simulink model "c00014M_harness"  (R2018a)
settings: Solver=FixedStepAuto  StartTime=0.0  StopTime=300  FixedStep=0.1  RelTol=1e-3
undefined symbols (not defined in the file): A1, hmax, PriorityTank, R1, R2, sigbuilder_block
(part 1 of 24)
settings Model: Creator=aarrieta  LastModifiedBy=umarkiegi

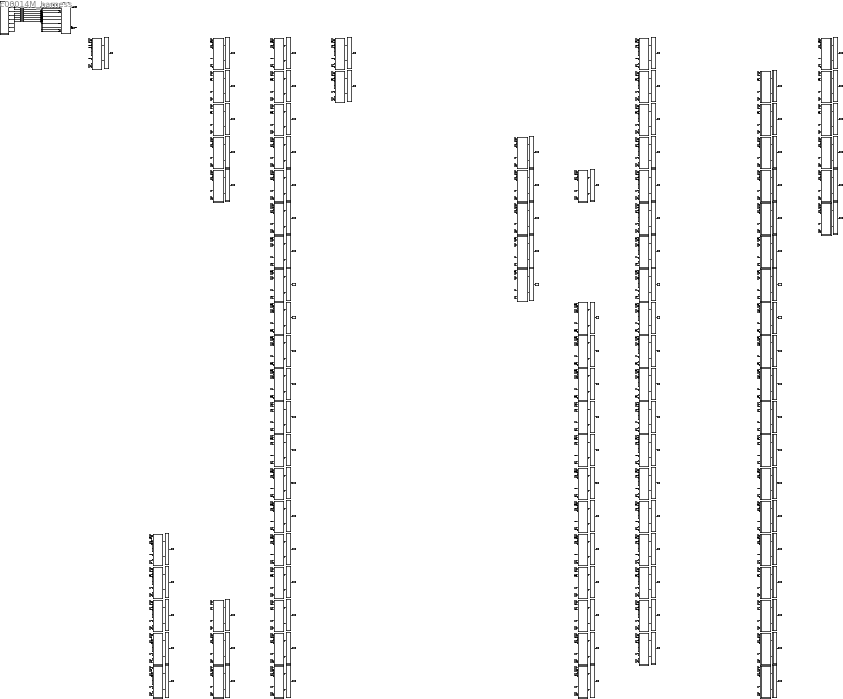
== system c00014M_harness ==
  CPSUT : Subsystem
  Eval : Subsystem
  Eval143 : Subsystem
  Eval144 : Subsystem
  Eval145 : Subsystem
  Eval146 : Subsystem
  Eval147 : Subsystem
  Eval164 : Subsystem
  Eval168 : Subsystem
  Eval169 : Subsystem
  Eval170 : Subsystem
  Eval171 : Subsystem
  Eval172 : Subsystem
  Eval173 : Subsystem
  Eval174 : Subsystem
  Eval175 : Subsystem
  Eval176 : Subsystem
  Eval177 : Subsystem
  Eval178 : Subsystem
  Eval179 : Subsystem
  Eval180 : Subsystem
  Eval181 : Subsystem
  Eval182 : Subsystem
  Eval183 : Subsystem
  Eval184 : Subsystem
  Eval185 : Subsystem
  Eval186 : Subsystem
  Eval187 : Subsystem
  Eval188 : Subsystem
  Eval189 : Subsystem
  Eval190 : Subsystem
  Eval191 : Subsystem
  Eval192 : Subsystem
  Eval193 : Subsystem
  Eval194 : Subsystem
  Eval195 : Subsystem
  Eval196 : Subsystem
  Eval197 : Subsystem
  Eval198 : Subsystem
  Eval221 : Subsystem
  Eval222 : Subsystem
  Eval223 : Subsystem
  Eval224 : Subsystem
  Eval225 : Subsystem
  Eval226 : Subsystem
  Eval227 : Subsystem
  Eval228 : Subsystem
  Eval229 : Subsystem
  Eval230 : Subsystem
  Eval231 : Subsystem
  Eval232 : Subsystem
  Eval233 : Subsystem
  Eval234 : Subsystem
  Eval235 : Subsystem
  Eval236 : Subsystem
  Eval237 : Subsystem
  Eval238 : Subsystem
  Eval239 : Subsystem
  Eval240 : Subsystem
  Eval241 : Subsystem
  Eval242 : Subsystem
  Eval243 : Subsystem
  Eval244 : Subsystem
  Eval245 : Subsystem
  Eval35 : Subsystem
  Eval36 : Subsystem
  Eval37 : Subsystem
  Eval38 : Subsystem
  Eval39 : Subsystem
  Eval40 : Subsystem
  Eval41 : Subsystem
  Eval42 : Subsystem
  Eval43 : Subsystem
  Eval44 : Subsystem
  Eval57 : Subsystem
  Eval58 : Subsystem
  Eval59 : Subsystem
  Eval60 : Subsystem
  Eval61 : Subsystem
  Eval62 : Subsystem
  Eval63 : Subsystem
  Eval64 : Subsystem
  Eval65 : Subsystem
  Eval66 : Subsystem
  Eval67 : Subsystem
  Eval68 : Subsystem
  Eval69 : Subsystem
  Eval70 : Subsystem
  Eval71 : Subsystem
  Eval72 : Subsystem
  Eval73 : Subsystem
  Eval74 : Subsystem
  Eval75 : Subsystem
  Eval76 : Subsystem
  Eval77 : Subsystem
  Eval78 : Subsystem
  Eval79 : Subsystem
  Eval80 : Subsystem
  Eval81 : Subsystem
  Inputs : Subsystem  Tag=STV Subsys  LoadFcn=sigbuilder_block('load');  StartFcn=sigbuilder_block('start');  StopFcn=sigbuilder_block('stop');  ClipboardFcn=sigbuilder_block('clipboard');  mask(Sigbuilder block){tuvar=[0:10]}
      mask init:
      | if ~strcmp(get_param(bdroot(gcb),'SimulationStatus'),'stopped'),tuvar = sigbuilder_block('maskInit'); end
      settings: CopyFcn=sigbuilder_block('copy');  DeleteFcn=sigbuilder_block('delete');  ModelCloseFcn=sigbuilder_block('modelClose');  PreSaveFcn=sigbuilder_block('preSave');  PauseFcn=sigbuilder_block('pause');  ContinueFcn=sigbuilder_block('continue');  NameChangeFcn=sigbuilder_block('namechange');  OpenFcn=sigbuilder_block('open',[276.75 163.5 675.75 486.75 ]);  CloseFcn=sigbuilder_block('close');
      mask Display: plot(0, 0, 100, 100,[2, 2, 32, 32, 2], [68, 8, 8, 68, 68],[32, 2], [38, 38], [32, 19, 2],[53, 60, 44], [32, 17, 17, 2],[16, 16, 31, 31]);txt = getActiveGroup(gcbh);text(2, 100, txt,'verticalAlignment', 'top');
  M001 : Subsystem
  M036 : Subsystem
  M037 : Subsystem
  M038 : Subsystem
  M039 : Subsystem
  M040 : Subsystem
  M041 : Subsystem
  M042 : Subsystem
  M043 : Subsystem
  M044 : Subsystem
  M045 : Subsystem
  M058 : Subsystem
  M059 : Subsystem
  M060 : Subsystem
  M061 : Subsystem
  M062 : Subsystem
  M063 : Subsystem
  M064 : Subsystem
  M065 : Subsystem
  M066 : Subsystem
  M067 : Subsystem
  M068 : Subsystem
  M069 : Subsystem
  M070 : Subsystem
  M071 : Subsystem
  M072 : Subsystem
  M073 : Subsystem
  M074 : Subsystem
  M075 : Subsystem
  M076 : Subsystem
  M077 : Subsystem
  M078 : Subsystem
  M079 : Subsystem
  M080 : Subsystem
  M081 : Subsystem
  M082 : Subsystem
  M144 : Subsystem
  M145 : Subsystem
  M146 : Subsystem
  M147 : Subsystem
  M148 : Subsystem
  M165 : Subsystem
  M169 : Subsystem
  M170 : Subsystem
  M171 : Subsystem
  M172 : Subsystem
  M173 : Subsystem
  M174 : Subsystem
  M175 : Subsystem
  M176 : Subsystem
  M177 : Subsystem
  M178 : Subsystem
  M179 : Subsystem
  M180 : Subsystem
  M181 : Subsystem
  M182 : Subsystem
  M183 : Subsystem
  M184 : Subsystem
  M185 : Subsystem
  M186 : Subsystem
  M187 : Subsystem
  M188 : Subsystem
  M189 : Subsystem
  M190 : Subsystem
  M191 : Subsystem
  M192 : Subsystem
  M193 : Subsystem
  M194 : Subsystem
  M195 : Subsystem
  M196 : Subsystem
  M197 : Subsystem
  M198 : Subsystem
  M199 : Subsystem
  M222 : Subsystem
  M223 : Subsystem
  M224 : Subsystem
  M225 : Subsystem
  M226 : Subsystem
  M227 : Subsystem
  M228 : Subsystem
  M229 : Subsystem
  M230 : Subsystem
  M231 : Subsystem
  M232 : Subsystem
  M233 : Subsystem
  M234 : Subsystem
  M235 : Subsystem
  M236 : Subsystem
  M237 : Subsystem
  M238 : Subsystem
  M239 : Subsystem
  M240 : Subsystem
  M241 : Subsystem
  M242 : Subsystem
  M243 : Subsystem
  M244 : Subsystem
  M245 : Subsystem
  M246 : Subsystem
  To Workspace : ToWorkspace  VariableName=mutant001  SampleTime=-1
  To Workspace143 : ToWorkspace  VariableName=mutant144  SampleTime=-1
  To Workspace144 : ToWorkspace  VariableName=mutant145  SampleTime=-1
  To Workspace145 : ToWorkspace  VariableName=mutant146  SampleTime=-1
  To Workspace146 : ToWorkspace  VariableName=mutant147  SampleTime=-1
  To Workspace147 : ToWorkspace  VariableName=mutant148  SampleTime=-1
  To Workspace164 : ToWorkspace  VariableName=mutant165  SampleTime=-1
  To Workspace168 : ToWorkspace  VariableName=mutant169  SampleTime=-1
  To Workspace169 : ToWorkspace  VariableName=mutant170  SampleTime=-1
  To Workspace170 : ToWorkspace  VariableName=mutant171  SampleTime=-1
  To Workspace171 : ToWorkspace  VariableName=mutant172  SampleTime=-1
  To Workspace172 : ToWorkspace  VariableName=mutant173  SampleTime=-1
  To Workspace173 : ToWorkspace  VariableName=mutant174  SampleTime=-1
  To Workspace174 : ToWorkspace  VariableName=mutant175  SampleTime=-1
  To Workspace175 : ToWorkspace  VariableName=mutant176  SampleTime=-1
  To Workspace176 : ToWorkspace  VariableName=mutant177  SampleTime=-1
  To Workspace177 : ToWorkspace  VariableName=mutant178  SampleTime=-1
  To Workspace178 : ToWorkspace  VariableName=mutant179  SampleTime=-1
  To Workspace179 : ToWorkspace  VariableName=mutant180  SampleTime=-1
  To Workspace180 : ToWorkspace  VariableName=mutant181  SampleTime=-1
  To Workspace181 : ToWorkspace  VariableName=mutant182  SampleTime=-1
  To Workspace182 : ToWorkspace  VariableName=mutant183  SampleTime=-1
  To Workspace183 : ToWorkspace  VariableName=mutant184  SampleTime=-1
  To Workspace184 : ToWorkspace  VariableName=mutant185  SampleTime=-1
  To Workspace185 : ToWorkspace  VariableName=mutant186  SampleTime=-1
  To Workspace186 : ToWorkspace  VariableName=mutant187  SampleTime=-1
  To Workspace187 : ToWorkspace  VariableName=mutant188  SampleTime=-1
  To Workspace188 : ToWorkspace  VariableName=mutant189  SampleTime=-1
  To Workspace189 : ToWorkspace  VariableName=mutant190  SampleTime=-1
  To Workspace190 : ToWorkspace  VariableName=mutant191  SampleTime=-1
  To Workspace191 : ToWorkspace  VariableName=mutant192  SampleTime=-1
  To Workspace192 : ToWorkspace  VariableName=mutant193  SampleTime=-1
  To Workspace193 : ToWorkspace  VariableName=mutant194  SampleTime=-1
  To Workspace194 : ToWorkspace  VariableName=mutant195  SampleTime=-1
  To Workspace195 : ToWorkspace  VariableName=mutant196  SampleTime=-1
  To Workspace196 : ToWorkspace  VariableName=mutant197  SampleTime=-1
  To Workspace197 : ToWorkspace  VariableName=mutant198  SampleTime=-1
  To Workspace198 : ToWorkspace  VariableName=mutant199  SampleTime=-1
  To Workspace221 : ToWorkspace  VariableName=mutant222  SampleTime=-1
  To Workspace222 : ToWorkspace  VariableName=mutant223  SampleTime=-1
  To Workspace223 : ToWorkspace  VariableName=mutant224  SampleTime=-1
  To Workspace224 : ToWorkspace  VariableName=mutant225  SampleTime=-1
  To Workspace225 : ToWorkspace  VariableName=mutant226  SampleTime=-1
  To Workspace226 : ToWorkspace  VariableName=mutant227  SampleTime=-1
  To Workspace227 : ToWorkspace  VariableName=mutant228  SampleTime=-1
  To Workspace228 : ToWorkspace  VariableName=mutant229  SampleTime=-1
  To Workspace229 : ToWorkspace  VariableName=mutant230  SampleTime=-1
  To Workspace230 : ToWorkspace  VariableName=mutant231  SampleTime=-1
  To Workspace231 : ToWorkspace  VariableName=mutant232  SampleTime=-1
  To Workspace232 : ToWorkspace  VariableName=mutant233  SampleTime=-1
  To Workspace233 : ToWorkspace  VariableName=mutant234  SampleTime=-1
  To Workspace234 : ToWorkspace  VariableName=mutant235  SampleTime=-1
  To Workspace235 : ToWorkspace  VariableName=mutant236  SampleTime=-1
  To Workspace236 : ToWorkspace  VariableName=mutant237  SampleTime=-1
  To Workspace237 : ToWorkspace  VariableName=mutant238  SampleTime=-1
  To Workspace238 : ToWorkspace  VariableName=mutant239  SampleTime=-1
  To Workspace239 : ToWorkspace  VariableName=mutant240  SampleTime=-1
  To Workspace240 : ToWorkspace  VariableName=mutant241  SampleTime=-1
  To Workspace241 : ToWorkspace  VariableName=mutant242  SampleTime=-1
  To Workspace242 : ToWorkspace  VariableName=mutant243  SampleTime=-1
  To Workspace243 : ToWorkspace  VariableName=mutant244  SampleTime=-1
  To Workspace244 : ToWorkspace  VariableName=mutant245  SampleTime=-1
  To Workspace245 : ToWorkspace  VariableName=mutant246  SampleTime=-1
  To Workspace35 : ToWorkspace  VariableName=mutant036  SampleTime=-1
  To Workspace36 : ToWorkspace  VariableName=mutant037  SampleTime=-1
  To Workspace37 : ToWorkspace  VariableName=mutant038  SampleTime=-1
  To Workspace38 : ToWorkspace  VariableName=mutant039  SampleTime=-1
  To Workspace39 : ToWorkspace  VariableName=mutant040  SampleTime=-1
  To Workspace40 : ToWorkspace  VariableName=mutant041  SampleTime=-1
  To Workspace41 : ToWorkspace  VariableName=mutant042  SampleTime=-1
  To Workspace42 : ToWorkspace  VariableName=mutant043  SampleTime=-1
  To Workspace43 : ToWorkspace  VariableName=mutant044  SampleTime=-1
  To Workspace44 : ToWorkspace  VariableName=mutant045  SampleTime=-1
  To Workspace57 : ToWorkspace  VariableName=mutant058  SampleTime=-1
  To Workspace58 : ToWorkspace  VariableName=mutant059  SampleTime=-1
  To Workspace59 : ToWorkspace  VariableName=mutant060  SampleTime=-1
  To Workspace60 : ToWorkspace  VariableName=mutant061  SampleTime=-1
  To Workspace61 : ToWorkspace  VariableName=mutant062  SampleTime=-1
  To Workspace62 : ToWorkspace  VariableName=mutant063  SampleTime=-1
  To Workspace63 : ToWorkspace  VariableName=mutant064  SampleTime=-1
  To Workspace64 : ToWorkspace  VariableName=mutant065  SampleTime=-1
  To Workspace65 : ToWorkspace  VariableName=mutant066  SampleTime=-1
  To Workspace66 : ToWorkspace  VariableName=mutant067  SampleTime=-1
  To Workspace67 : ToWorkspace  VariableName=mutant068  SampleTime=-1
  To Workspace68 : ToWorkspace  VariableName=mutant069  SampleTime=-1
  To Workspace69 : ToWorkspace  VariableName=mutant070  SampleTime=-1
  To Workspace70 : ToWorkspace  VariableName=mutant071  SampleTime=-1
  To Workspace71 : ToWorkspace  VariableName=mutant072  SampleTime=-1
  To Workspace72 : ToWorkspace  VariableName=mutant073  SampleTime=-1
  To Workspace73 : ToWorkspace  VariableName=mutant074  SampleTime=-1
  To Workspace74 : ToWorkspace  VariableName=mutant075  SampleTime=-1
  To Workspace75 : ToWorkspace  VariableName=mutant076  SampleTime=-1
  To Workspace76 : ToWorkspace  VariableName=mutant077  SampleTime=-1
  To Workspace77 : ToWorkspace  VariableName=mutant078  SampleTime=-1
  To Workspace78 : ToWorkspace  VariableName=mutant079  SampleTime=-1
  To Workspace79 : ToWorkspace  VariableName=mutant080  SampleTime=-1
  To Workspace80 : ToWorkspace  VariableName=mutant081  SampleTime=-1
  To Workspace81 : ToWorkspace  VariableName=mutant082  SampleTime=-1
  dtc_CT1 : DataTypeConversion
  dtc_CT3 : DataTypeConversion
  dtc_E1 : DataTypeConversion
  dtc_EB1 : DataTypeConversion
  dtc_EB3 : DataTypeConversion
  dtc_F1 : DataTypeConversion
  dtc_T1 : DataTypeConversion
  dtc_T3 : DataTypeConversion
  LL1 : Outport
  LL3 : Outport  Port=2
  tag scope: out1=global, out3=global
  wires:
  CPSUT/1(LL1) -> [out1], LL1/1
  CPSUT/2(LL3) -> [out3], LL3/1
  [in1] -> M001/1(CT1)
  [in2] -> M001/2(F1)
  [in3] -> M001/3(E1)
  [in5] -> M001/4(T1)
  [in6] -> M001/5(EB1)
  [in13] -> M001/6(CT3)
  [in17] -> M001/7(T3)
  [in18] -> M001/8(EB3)
  Eval/1(Out1) -> To Workspace/1
  M001/1(LL1) -> Eval/1(In1)
  M001/2(LL3) -> Eval/2(In3)
  [in1] -> M036/1(CT1)
  [in2] -> M036/2(F1)
  [in3] -> M036/3(E1)
  [in5] -> M036/4(T1)
  [in6] -> M036/5(EB1)
  [in13] -> M036/6(CT3)
  [in17] -> M036/7(T3)
  [in18] -> M036/8(EB3)
  M036/1(LL1) -> Eval35/1(In1)
  M036/2(LL3) -> Eval35/2(In3)
  Eval35/1(Out1) -> To Workspace35/1
  [in1] -> M037/1(CT1)
  [in2] -> M037/2(F1)
  [in3] -> M037/3(E1)
  [in5] -> M037/4(T1)
  [in6] -> M037/5(EB1)
  [in13] -> M037/6(CT3)
  [in17] -> M037/7(T3)
  [in18] -> M037/8(EB3)
  M037/1(LL1) -> Eval36/1(In1)
  M037/2(LL3) -> Eval36/2(In3)
  Eval36/1(Out1) -> To Workspace36/1
  [in1] -> M038/1(CT1)
  [in2] -> M038/2(F1)
  [in3] -> M038/3(E1)
  [in5] -> M038/4(T1)
  [in6] -> M038/5(EB1)
  [in13] -> M038/6(CT3)
  [in17] -> M038/7(T3)
  [in18] -> M038/8(EB3)
  M038/1(LL1) -> Eval37/1(In1)
  M038/2(LL3) -> Eval37/2(In3)
  Eval37/1(Out1) -> To Workspace37/1
  [in1] -> M039/1(CT1)
  [in2] -> M039/2(F1)
  [in3] -> M039/3(E1)
  [in5] -> M039/4(T1)
  [in6] -> M039/5(EB1)
  [in13] -> M039/6(CT3)
  [in17] -> M039/7(T3)
  [in18] -> M039/8(EB3)
  M039/1(LL1) -> Eval38/1(In1)
  M039/2(LL3) -> Eval38/2(In3)
  Eval38/1(Out1) -> To Workspace38/1
  [in1] -> M040/1(CT1)
  [in2] -> M040/2(F1)
  [in3] -> M040/3(E1)
  [in5] -> M040/4(T1)
  [in6] -> M040/5(EB1)
  [in13] -> M040/6(CT3)
  [in17] -> M040/7(T3)
  [in18] -> M040/8(EB3)
  M040/1(LL1) -> Eval39/1(In1)
  M040/2(LL3) -> Eval39/2(In3)
  Eval39/1(Out1) -> To Workspace39/1
  [in1] -> M041/1(CT1)
  [in2] -> M041/2(F1)
  [in3] -> M041/3(E1)
  [in5] -> M041/4(T1)
  [in6] -> M041/5(EB1)
  [in13] -> M041/6(CT3)
  [in17] -> M041/7(T3)
  [in18] -> M041/8(EB3)
  M041/1(LL1) -> Eval40/1(In1)
  M041/2(LL3) -> Eval40/2(In3)
  Eval40/1(Out1) -> To Workspace40/1
  [in1] -> M042/1(CT1)
  [in2] -> M042/2(F1)
  [in3] -> M042/3(E1)
  [in5] -> M042/4(T1)
  [in6] -> M042/5(EB1)
  [in13] -> M042/6(CT3)
  [in17] -> M042/7(T3)
  [in18] -> M042/8(EB3)
  M042/1(LL1) -> Eval41/1(In1)
  M042/2(LL3) -> Eval41/2(In3)
  Eval41/1(Out1) -> To Workspace41/1
  [in1] -> M043/1(CT1)
  [in2] -> M043/2(F1)
  [in3] -> M043/3(E1)
  [in5] -> M043/4(T1)
  [in6] -> M043/5(EB1)
  [in13] -> M043/6(CT3)
  [in17] -> M043/7(T3)
  [in18] -> M043/8(EB3)
  M043/1(LL1) -> Eval42/1(In1)
  M043/2(LL3) -> Eval42/2(In3)
  Eval42/1(Out1) -> To Workspace42/1
  [in1] -> M044/1(CT1)
  [in2] -> M044/2(F1)
  [in3] -> M044/3(E1)
  [in5] -> M044/4(T1)
  [in6] -> M044/5(EB1)
  [in13] -> M044/6(CT3)
  [in17] -> M044/7(T3)
  [in18] -> M044/8(EB3)
  M044/1(LL1) -> Eval43/1(In1)
  M044/2(LL3) -> Eval43/2(In3)
  Eval43/1(Out1) -> To Workspace43/1
  [in1] -> M045/1(CT1)
  [in2] -> M045/2(F1)
  [in3] -> M045/3(E1)
  [in5] -> M045/4(T1)
  [in6] -> M045/5(EB1)
  [in13] -> M045/6(CT3)
  [in17] -> M045/7(T3)
  [in18] -> M045/8(EB3)
  M045/1(LL1) -> Eval44/1(In1)
  M045/2(LL3) -> Eval44/2(In3)
  Eval44/1(Out1) -> To Workspace44/1
  [in1] -> M058/1(CT1)
  [in2] -> M058/2(F1)
  [in3] -> M058/3(E1)
  [in5] -> M058/4(T1)
  [in6] -> M058/5(EB1)
  [in13] -> M058/6(CT3)
  [in17] -> M058/7(T3)
  [in18] -> M058/8(EB3)
  M058/1(LL1) -> Eval57/1(In1)
  M058/2(LL3) -> Eval57/2(In3)
  Eval57/1(Out1) -> To Workspace57/1
  [in1] -> M059/1(CT1)
  [in2] -> M059/2(F1)
  [in3] -> M059/3(E1)
  [in5] -> M059/4(T1)
  [in6] -> M059/5(EB1)
  [in13] -> M059/6(CT3)
  [in17] -> M059/7(T3)
  [in18] -> M059/8(EB3)
  M059/1(LL1) -> Eval58/1(In1)
  M059/2(LL3) -> Eval58/2(In3)
  Eval58/1(Out1) -> To Workspace58/1
  [in1] -> M060/1(CT1)
  [in2] -> M060/2(F1)
  [in3] -> M060/3(E1)
  [in5] -> M060/4(T1)
  [in6] -> M060/5(EB1)
  [in13] -> M060/6(CT3)
  [in17] -> M060/7(T3)
  [in18] -> M060/8(EB3)
  M060/1(LL1) -> Eval59/1(In1)
  M060/2(LL3) -> Eval59/2(In3)
  Eval59/1(Out1) -> To Workspace59/1
  [in1] -> M061/1(CT1)
  [in2] -> M061/2(F1)
  [in3] -> M061/3(E1)
  [in5] -> M061/4(T1)
  [in6] -> M061/5(EB1)
  [in13] -> M061/6(CT3)
  [in17] -> M061/7(T3)
  [in18] -> M061/8(EB3)
  M061/1(LL1) -> Eval60/1(In1)
  M061/2(LL3) -> Eval60/2(In3)
  Eval60/1(Out1) -> To Workspace60/1
  [in1] -> M062/1(CT1)
  [in2] -> M062/2(F1)
  [in3] -> M062/3(E1)
  [in5] -> M062/4(T1)
  [in6] -> M062/5(EB1)
  [in13] -> M062/6(CT3)
  [in17] -> M062/7(T3)
  [in18] -> M062/8(EB3)
  M062/1(LL1) -> Eval61/1(In1)
  M062/2(LL3) -> Eval61/2(In3)
  Eval61/1(Out1) -> To Workspace61/1
  [in1] -> M063/1(CT1)
  [in2] -> M063/2(F1)
  [in3] -> M063/3(E1)
  [in5] -> M063/4(T1)
  [in6] -> M063/5(EB1)
  [in13] -> M063/6(CT3)
  [in17] -> M063/7(T3)
  [in18] -> M063/8(EB3)
  M063/1(LL1) -> Eval62/1(In1)
  M063/2(LL3) -> Eval62/2(In3)
  Eval62/1(Out1) -> To Workspace62/1
  [in1] -> M064/1(CT1)
  [in2] -> M064/2(F1)
  [in3] -> M064/3(E1)
  [in5] -> M064/4(T1)
  [in6] -> M064/5(EB1)
  [in13] -> M064/6(CT3)
  [in17] -> M064/7(T3)
  [in18] -> M064/8(EB3)
  M064/1(LL1) -> Eval63/1(In1)
  M064/2(LL3) -> Eval63/2(In3)
  Eval63/1(Out1) -> To Workspace63/1
  [in1] -> M065/1(CT1)
  [in2] -> M065/2(F1)
  [in3] -> M065/3(E1)
  [in5] -> M065/4(T1)
  [in6] -> M065/5(EB1)
  [in13] -> M065/6(CT3)
  [in17] -> M065/7(T3)
  [in18] -> M065/8(EB3)
  M065/1(LL1) -> Eval64/1(In1)
  M065/2(LL3) -> Eval64/2(In3)
  Eval64/1(Out1) -> To Workspace64/1
  [in1] -> M066/1(CT1)
  [in2] -> M066/2(F1)
  [in3] -> M066/3(E1)
  [in5] -> M066/4(T1)
  [in6] -> M066/5(EB1)
  [in13] -> M066/6(CT3)
  [in17] -> M066/7(T3)
  [in18] -> M066/8(EB3)
  M066/1(LL1) -> Eval65/1(In1)
  M066/2(LL3) -> Eval65/2(In3)
  Eval65/1(Out1) -> To Workspace65/1
  [in1] -> M067/1(CT1)
  [in2] -> M067/2(F1)
  [in3] -> M067/3(E1)
  [in5] -> M067/4(T1)
  [in6] -> M067/5(EB1)
  [in13] -> M067/6(CT3)
  [in17] -> M067/7(T3)
  [in18] -> M067/8(EB3)
  M067/1(LL1) -> Eval66/1(In1)
  M067/2(LL3) -> Eval66/2(In3)
  Eval66/1(Out1) -> To Workspace66/1
  [in1] -> M068/1(CT1)
  [in2] -> M068/2(F1)
  [in3] -> M068/3(E1)
  [in5] -> M068/4(T1)
  [in6] -> M068/5(EB1)
  [in13] -> M068/6(CT3)
  [in17] -> M068/7(T3)
  [in18] -> M068/8(EB3)
  M068/1(LL1) -> Eval67/1(In1)
  M068/2(LL3) -> Eval67/2(In3)
  Eval67/1(Out1) -> To Workspace67/1
  [in1] -> M069/1(CT1)
  [in2] -> M069/2(F1)
  [in3] -> M069/3(E1)
  [in5] -> M069/4(T1)
  [in6] -> M069/5(EB1)
  [in13] -> M069/6(CT3)
  [in17] -> M069/7(T3)
  [in18] -> M069/8(EB3)
  M069/1(LL1) -> Eval68/1(In1)
  M069/2(LL3) -> Eval68/2(In3)
  Eval68/1(Out1) -> To Workspace68/1
  [in1] -> M070/1(CT1)
  [in2] -> M070/2(F1)
  [in3] -> M070/3(E1)
  [in5] -> M070/4(T1)
  [in6] -> M070/5(EB1)
  [in13] -> M070/6(CT3)
  [in17] -> M070/7(T3)
  [in18] -> M070/8(EB3)
  M070/1(LL1) -> Eval69/1(In1)
  M070/2(LL3) -> Eval69/2(In3)
  Eval69/1(Out1) -> To Workspace69/1
  [in1] -> M071/1(CT1)
  [in2] -> M071/2(F1)
  [in3] -> M071/3(E1)
  [in5] -> M071/4(T1)
  [in6] -> M071/5(EB1)
  [in13] -> M071/6(CT3)
  [in17] -> M071/7(T3)
  [in18] -> M071/8(EB3)
  M071/1(LL1) -> Eval70/1(In1)
  M071/2(LL3) -> Eval70/2(In3)
  Eval70/1(Out1) -> To Workspace70/1
  [in1] -> M072/1(CT1)
  [in2] -> M072/2(F1)
  [in3] -> M072/3(E1)
  [in5] -> M072/4(T1)
  [in6] -> M072/5(EB1)
  [in13] -> M072/6(CT3)
  [in17] -> M072/7(T3)
  [in18] -> M072/8(EB3)
  M072/1(LL1) -> Eval71/1(In1)
  M072/2(LL3) -> Eval71/2(In3)
  Eval71/1(Out1) -> To Workspace71/1
  [in1] -> M073/1(CT1)
  [in2] -> M073/2(F1)
  [in3] -> M073/3(E1)
  [in5] -> M073/4(T1)
  [in6] -> M073/5(EB1)
  [in13] -> M073/6(CT3)
  [in17] -> M073/7(T3)
  [in18] -> M073/8(EB3)
  M073/1(LL1) -> Eval72/1(In1)
  M073/2(LL3) -> Eval72/2(In3)
  Eval72/1(Out1) -> To Workspace72/1
  [in1] -> M074/1(CT1)
  [in2] -> M074/2(F1)
  [in3] -> M074/3(E1)
  [in5] -> M074/4(T1)
  [in6] -> M074/5(EB1)
  [in13] -> M074/6(CT3)
  [in17] -> M074/7(T3)
  [in18] -> M074/8(EB3)
  M074/1(LL1) -> Eval73/1(In1)
  M074/2(LL3) -> Eval73/2(In3)
  Eval73/1(Out1) -> To Workspace73/1
  [in1] -> M075/1(CT1)
  [in2] -> M075/2(F1)
  [in3] -> M075/3(E1)
  [in5] -> M075/4(T1)
  [in6] -> M075/5(EB1)
  [in13] -> M075/6(CT3)
  [in17] -> M075/7(T3)
  [in18] -> M075/8(EB3)
  M075/1(LL1) -> Eval74/1(In1)
  M075/2(LL3) -> Eval74/2(In3)
  Eval74/1(Out1) -> To Workspace74/1
  [in1] -> M076/1(CT1)
  [in2] -> M076/2(F1)
  [in3] -> M076/3(E1)
  [in5] -> M076/4(T1)
  [in6] -> M076/5(EB1)
  [in13] -> M076/6(CT3)
  [in17] -> M076/7(T3)
  [in18] -> M076/8(EB3)
  M076/1(LL1) -> Eval75/1(In1)
  M076/2(LL3) -> Eval75/2(In3)
  Eval75/1(Out1) -> To Workspace75/1
  [in1] -> M077/1(CT1)
  [in2] -> M077/2(F1)
  [in3] -> M077/3(E1)
  [in5] -> M077/4(T1)
  [in6] -> M077/5(EB1)
  [in13] -> M077/6(CT3)
  [in17] -> M077/7(T3)
  [in18] -> M077/8(EB3)
  M077/1(LL1) -> Eval76/1(In1)
  M077/2(LL3) -> Eval76/2(In3)
  Eval76/1(Out1) -> To Workspace76/1
  [in1] -> M078/1(CT1)
  [in2] -> M078/2(F1)
  [in3] -> M078/3(E1)
  [in5] -> M078/4(T1)
  [in6] -> M078/5(EB1)
  [in13] -> M078/6(CT3)
  [in17] -> M078/7(T3)
  [in18] -> M078/8(EB3)
  M078/1(LL1) -> Eval77/1(In1)
  M078/2(LL3) -> Eval77/2(In3)
  Eval77/1(Out1) -> To Workspace77/1
  [in1] -> M079/1(CT1)
  [in2] -> M079/2(F1)
  [in3] -> M079/3(E1)
  [in5] -> M079/4(T1)
  [in6] -> M079/5(EB1)
  [in13] -> M079/6(CT3)
  [in17] -> M079/7(T3)
  [in18] -> M079/8(EB3)
  M079/1(LL1) -> Eval78/1(In1)
  M079/2(LL3) -> Eval78/2(In3)
  Eval78/1(Out1) -> To Workspace78/1
  [in1] -> M080/1(CT1)
  [in2] -> M080/2(F1)
  [in3] -> M080/3(E1)
  [in5] -> M080/4(T1)
  [in6] -> M080/5(EB1)
  [in13] -> M080/6(CT3)
  [in17] -> M080/7(T3)
  [in18] -> M080/8(EB3)
  M080/1(LL1) -> Eval79/1(In1)
  M080/2(LL3) -> Eval79/2(In3)
  Eval79/1(Out1) -> To Workspace79/1
  [in1] -> M081/1(CT1)
  [in2] -> M081/2(F1)
  [in3] -> M081/3(E1)
  [in5] -> M081/4(T1)
  [in6] -> M081/5(EB1)
  [in13] -> M081/6(CT3)
  [in17] -> M081/7(T3)
  [in18] -> M081/8(EB3)
  M081/1(LL1) -> Eval80/1(In1)
  M081/2(LL3) -> Eval80/2(In3)
  Eval80/1(Out1) -> To Workspace80/1
  [in1] -> M082/1(CT1)
  [in2] -> M082/2(F1)
  [in3] -> M082/3(E1)
  [in5] -> M082/4(T1)
  [in6] -> M082/5(EB1)
  [in13] -> M082/6(CT3)
  [in17] -> M082/7(T3)
  [in18] -> M082/8(EB3)
  M082/1(LL1) -> Eval81/1(In1)
  M082/2(LL3) -> Eval81/2(In3)
  Eval81/1(Out1) -> To Workspace81/1
  [in1] -> M144/1(CT1)
  [in2] -> M144/2(F1)
  [in3] -> M144/3(E1)
  [in5] -> M144/4(T1)
  [in6] -> M144/5(EB1)
  [in13] -> M144/6(CT3)
  [in17] -> M144/7(T3)
  [in18] -> M144/8(EB3)
  M144/1(LL1) -> Eval143/1(In1)
  M144/2(LL3) -> Eval143/2(In3)
  Eval143/1(Out1) -> To Workspace143/1
  [in1] -> M145/1(CT1)
  [in2] -> M145/2(F1)
  [in3] -> M145/3(E1)
  [in5] -> M145/4(T1)
  [in6] -> M145/5(EB1)
  [in13] -> M145/6(CT3)
  [in17] -> M145/7(T3)
  [in18] -> M145/8(EB3)
  M145/1(LL1) -> Eval144/1(In1)
  M145/2(LL3) -> Eval144/2(In3)
  Eval144/1(Out1) -> To Workspace144/1
  [in1] -> M146/1(CT1)
  [in2] -> M146/2(F1)
  [in3] -> M146/3(E1)
  [in5] -> M146/4(T1)
  [in6] -> M146/5(EB1)
  [in13] -> M146/6(CT3)
  [in17] -> M146/7(T3)
  [in18] -> M146/8(EB3)
  M146/1(LL1) -> Eval145/1(In1)
  M146/2(LL3) -> Eval145/2(In3)
  Eval145/1(Out1) -> To Workspace145/1
  [in1] -> M147/1(CT1)
  [in2] -> M147/2(F1)
  [in3] -> M147/3(E1)
  [in5] -> M147/4(T1)
  [in6] -> M147/5(EB1)
  [in13] -> M147/6(CT3)
  [in17] -> M147/7(T3)
  [in18] -> M147/8(EB3)
  M147/1(LL1) -> Eval146/1(In1)
  M147/2(LL3) -> Eval146/2(In3)
  Eval146/1(Out1) -> To Workspace146/1
  [in1] -> M148/1(CT1)
  [in2] -> M148/2(F1)
  [in3] -> M148/3(E1)
  [in5] -> M148/4(T1)
  [in6] -> M148/5(EB1)
  [in13] -> M148/6(CT3)
  [in17] -> M148/7(T3)
  [in18] -> M148/8(EB3)
  M148/1(LL1) -> Eval147/1(In1)
  M148/2(LL3) -> Eval147/2(In3)
  Eval147/1(Out1) -> To Workspace147/1
  [in1] -> M165/1(CT1)
  [in2] -> M165/2(F1)
  [in3] -> M165/3(E1)
  [in5] -> M165/4(T1)
  [in6] -> M165/5(EB1)
  [in13] -> M165/6(CT3)
  [in17] -> M165/7(T3)
  [in18] -> M165/8(EB3)
  M165/1(LL1) -> Eval164/1(In1)
  M165/2(LL3) -> Eval164/2(In3)
  Eval164/1(Out1) -> To Workspace164/1
  [in1] -> M169/1(CT1)
  [in2] -> M169/2(F1)
  [in3] -> M169/3(E1)
  [in5] -> M169/4(T1)
  [in6] -> M169/5(EB1)
  [in13] -> M169/6(CT3)
  [in17] -> M169/7(T3)
  [in18] -> M169/8(EB3)
  M169/1(LL1) -> Eval168/1(In1)
  M169/2(LL3) -> Eval168/2(In3)
  Eval168/1(Out1) -> To Workspace168/1
  [in1] -> M170/1(CT1)
  [in2] -> M170/2(F1)
  [in3] -> M170/3(E1)
  [in5] -> M170/4(T1)
  [in6] -> M170/5(EB1)
  [in13] -> M170/6(CT3)
  [in17] -> M170/7(T3)
  [in18] -> M170/8(EB3)
  M170/1(LL1) -> Eval169/1(In1)
  M170/2(LL3) -> Eval169/2(In3)
  Eval169/1(Out1) -> To Workspace169/1
  [in1] -> M171/1(CT1)
  [in2] -> M171/2(F1)
  [in3] -> M171/3(E1)
  [in5] -> M171/4(T1)
  [in6] -> M171/5(EB1)
  [in13] -> M171/6(CT3)
  [in17] -> M171/7(T3)
  [in18] -> M171/8(EB3)
  M171/1(LL1) -> Eval170/1(In1)
  M171/2(LL3) -> Eval170/2(In3)
  Eval170/1(Out1) -> To Workspace170/1
  [in1] -> M172/1(CT1)
  [in2] -> M172/2(F1)
  [in3] -> M172/3(E1)
  [in5] -> M172/4(T1)
  [in6] -> M172/5(EB1)
  [in13] -> M172/6(CT3)
  [in17] -> M172/7(T3)
  [in18] -> M172/8(EB3)
  M172/1(LL1) -> Eval171/1(In1)
  M172/2(LL3) -> Eval171/2(In3)
  Eval171/1(Out1) -> To Workspace171/1
  [in1] -> M173/1(CT1)
  [in2] -> M173/2(F1)
  [in3] -> M173/3(E1)
  [in5] -> M173/4(T1)
  [in6] -> M173/5(EB1)
  [in13] -> M173/6(CT3)
  [in17] -> M173/7(T3)
  [in18] -> M173/8(EB3)
  M173/1(LL1) -> Eval172/1(In1)
  M173/2(LL3) -> Eval172/2(In3)
  Eval172/1(Out1) -> To Workspace172/1
  [in1] -> M174/1(CT1)
  [in2] -> M174/2(F1)
  [in3] -> M174/3(E1)
  [in5] -> M174/4(T1)
  [in6] -> M174/5(EB1)
  [in13] -> M174/6(CT3)
  [in17] -> M174/7(T3)
  [in18] -> M174/8(EB3)
  M174/1(LL1) -> Eval173/1(In1)
  M174/2(LL3) -> Eval173/2(In3)
  Eval173/1(Out1) -> To Workspace173/1
  [in1] -> M175/1(CT1)
  [in2] -> M175/2(F1)
  [in3] -> M175/3(E1)
  [in5] -> M175/4(T1)
  [in6] -> M175/5(EB1)
  [in13] -> M175/6(CT3)
  [in17] -> M175/7(T3)
  [in18] -> M175/8(EB3)
  M175/1(LL1) -> Eval174/1(In1)
  M175/2(LL3) -> Eval174/2(In3)
  Eval174/1(Out1) -> To Workspace174/1
  [in1] -> M176/1(CT1)
  [in2] -> M176/2(F1)
  [in3] -> M176/3(E1)
  [in5] -> M176/4(T1)
  [in6] -> M176/5(EB1)
  [in13] -> M176/6(CT3)
  [in17] -> M176/7(T3)
  [in18] -> M176/8(EB3)
  M176/1(LL1) -> Eval175/1(In1)
  M176/2(LL3) -> Eval175/2(In3)
  Eval175/1(Out1) -> To Workspace175/1
  [in1] -> M177/1(CT1)
  [in2] -> M177/2(F1)
  [in3] -> M177/3(E1)
  [in5] -> M177/4(T1)
  [in6] -> M177/5(EB1)
  [in13] -> M177/6(CT3)
  [in17] -> M177/7(T3)
  [in18] -> M177/8(EB3)
  M177/1(LL1) -> Eval176/1(In1)
  M177/2(LL3) -> Eval176/2(In3)
  Eval176/1(Out1) -> To Workspace176/1
  [in1] -> M178/1(CT1)
  [in2] -> M178/2(F1)
  [in3] -> M178/3(E1)
  [in5] -> M178/4(T1)
  [in6] -> M178/5(EB1)
  [in13] -> M178/6(CT3)
  [in17] -> M178/7(T3)
  [in18] -> M178/8(EB3)
  M178/1(LL1) -> Eval177/1(In1)
  M178/2(LL3) -> Eval177/2(In3)
  Eval177/1(Out1) -> To Workspace177/1
  [in1] -> M179/1(CT1)
  [in2] -> M179/2(F1)
  [in3] -> M179/3(E1)
  [in5] -> M179/4(T1)
  [in6] -> M179/5(EB1)
  [in13] -> M179/6(CT3)
  [in17] -> M179/7(T3)
  [in18] -> M179/8(EB3)
  M179/1(LL1) -> Eval178/1(In1)
  M179/2(LL3) -> Eval178/2(In3)
  Eval178/1(Out1) -> To Workspace178/1
  [in1] -> M180/1(CT1)
  [in2] -> M180/2(F1)
  [in3] -> M180/3(E1)
  [in5] -> M180/4(T1)
  [in6] -> M180/5(EB1)
  [in13] -> M180/6(CT3)
  [in17] -> M180/7(T3)
  [in18] -> M180/8(EB3)
  M180/1(LL1) -> Eval179/1(In1)
  M180/2(LL3) -> Eval179/2(In3)
  Eval179/1(Out1) -> To Workspace179/1
  [in1] -> M181/1(CT1)
  [in2] -> M181/2(F1)
  [in3] -> M181/3(E1)
  [in5] -> M181/4(T1)
  [in6] -> M181/5(EB1)
  [in13] -> M181/6(CT3)
  [in17] -> M181/7(T3)
  [in18] -> M181/8(EB3)
  M181/1(LL1) -> Eval180/1(In1)
  M181/2(LL3) -> Eval180/2(In3)
  Eval180/1(Out1) -> To Workspace180/1
  [in1] -> M182/1(CT1)
  [in2] -> M182/2(F1)
  [in3] -> M182/3(E1)
  [in5] -> M182/4(T1)
  [in6] -> M182/5(EB1)
  [in13] -> M182/6(CT3)
  [in17] -> M182/7(T3)
  [in18] -> M182/8(EB3)
  M182/1(LL1) -> Eval181/1(In1)
  M182/2(LL3) -> Eval181/2(In3)
  Eval181/1(Out1) -> To Workspace181/1
  [in1] -> M183/1(CT1)
  [in2] -> M183/2(F1)
  [in3] -> M183/3(E1)
  [in5] -> M183/4(T1)
  [in6] -> M183/5(EB1)
  [in13] -> M183/6(CT3)
  [in17] -> M183/7(T3)
  [in18] -> M183/8(EB3)
  M183/1(LL1) -> Eval182/1(In1)
  M183/2(LL3) -> Eval182/2(In3)
  Eval182/1(Out1) -> To Workspace182/1
  [in1] -> M184/1(CT1)
  [in2] -> M184/2(F1)
  [in3] -> M184/3(E1)
  [in5] -> M184/4(T1)
  [in6] -> M184/5(EB1)
  [in13] -> M184/6(CT3)
  [in17] -> M184/7(T3)
  [in18] -> M184/8(EB3)
  M184/1(LL1) -> Eval183/1(In1)
  M184/2(LL3) -> Eval183/2(In3)
  Eval183/1(Out1) -> To Workspace183/1
  [in1] -> M185/1(CT1)
  [in2] -> M185/2(F1)
  [in3] -> M185/3(E1)
  [in5] -> M185/4(T1)
  [in6] -> M185/5(EB1)
  [in13] -> M185/6(CT3)
  [in17] -> M185/7(T3)
  [in18] -> M185/8(EB3)
  M185/1(LL1) -> Eval184/1(In1)
  M185/2(LL3) -> Eval184/2(In3)
  Eval184/1(Out1) -> To Workspace184/1
  [in1] -> M186/1(CT1)
  [in2] -> M186/2(F1)
  [in3] -> M186/3(E1)
  [in5] -> M186/4(T1)
  [in6] -> M186/5(EB1)
  [in13] -> M186/6(CT3)
  [in17] -> M186/7(T3)
  [in18] -> M186/8(EB3)
  M186/1(LL1) -> Eval185/1(In1)
  M186/2(LL3) -> Eval185/2(In3)
  Eval185/1(Out1) -> To Workspace185/1
  [in1] -> M187/1(CT1)
  [in2] -> M187/2(F1)
  [in3] -> M187/3(E1)
  [in5] -> M187/4(T1)
  [in6] -> M187/5(EB1)
  [in13] -> M187/6(CT3)
  [in17] -> M187/7(T3)
  [in18] -> M187/8(EB3)
  M187/1(LL1) -> Eval186/1(In1)
  M187/2(LL3) -> Eval186/2(In3)
  Eval186/1(Out1) -> To Workspace186/1
  [in1] -> M188/1(CT1)
  [in2] -> M188/2(F1)
  [in3] -> M188/3(E1)
  [in5] -> M188/4(T1)
  [in6] -> M188/5(EB1)
  [in13] -> M188/6(CT3)
  [in17] -> M188/7(T3)
  [in18] -> M188/8(EB3)
  M188/1(LL1) -> Eval187/1(In1)
  M188/2(LL3) -> Eval187/2(In3)
  Eval187/1(Out1) -> To Workspace187/1
  [in1] -> M189/1(CT1)
  [in2] -> M189/2(F1)
  [in3] -> M189/3(E1)
  [in5] -> M189/4(T1)
  [in6] -> M189/5(EB1)
  [in13] -> M189/6(CT3)
  [in17] -> M189/7(T3)
  [in18] -> M189/8(EB3)
  M189/1(LL1) -> Eval188/1(In1)
  M189/2(LL3) -> Eval188/2(In3)
  Eval188/1(Out1) -> To Workspace188/1
  [in1] -> M190/1(CT1)
  [in2] -> M190/2(F1)
  [in3] -> M190/3(E1)
  [in5] -> M190/4(T1)
  [in6] -> M190/5(EB1)
  [in13] -> M190/6(CT3)
  [in17] -> M190/7(T3)
  [in18] -> M190/8(EB3)
  M190/1(LL1) -> Eval189/1(In1)
  M190/2(LL3) -> Eval189/2(In3)
  Eval189/1(Out1) -> To Workspace189/1
  [in1] -> M191/1(CT1)
  [in2] -> M191/2(F1)
  [in3] -> M191/3(E1)
  [in5] -> M191/4(T1)
  [in6] -> M191/5(EB1)
  [in13] -> M191/6(CT3)
  [in17] -> M191/7(T3)
  [in18] -> M191/8(EB3)
  M191/1(LL1) -> Eval190/1(In1)
  M191/2(LL3) -> Eval190/2(In3)
  Eval190/1(Out1) -> To Workspace190/1
  [in1] -> M192/1(CT1)
  [in2] -> M192/2(F1)
  [in3] -> M192/3(E1)
  [in5] -> M192/4(T1)
  [in6] -> M192/5(EB1)
  [in13] -> M192/6(CT3)
  [in17] -> M192/7(T3)
  [in18] -> M192/8(EB3)
  M192/1(LL1) -> Eval191/1(In1)
  M192/2(LL3) -> Eval191/2(In3)
  Eval191/1(Out1) -> To Workspace191/1
  [in1] -> M193/1(CT1)
  [in2] -> M193/2(F1)
  [in3] -> M193/3(E1)
  [in5] -> M193/4(T1)
  [in6] -> M193/5(EB1)
  [in13] -> M193/6(CT3)
  [in17] -> M193/7(T3)
  [in18] -> M193/8(EB3)
  M193/1(LL1) -> Eval192/1(In1)
  M193/2(LL3) -> Eval192/2(In3)
  Eval192/1(Out1) -> To Workspace192/1
  [in1] -> M194/1(CT1)
  [in2] -> M194/2(F1)
  [in3] -> M194/3(E1)
  [in5] -> M194/4(T1)
  [in6] -> M194/5(EB1)
  [in13] -> M194/6(CT3)
  [in17] -> M194/7(T3)
  [in18] -> M194/8(EB3)
  M194/1(LL1) -> Eval193/1(In1)
  M194/2(LL3) -> Eval193/2(In3)
  Eval193/1(Out1) -> To Workspace193/1
  [in1] -> M195/1(CT1)
  [in2] -> M195/2(F1)
  [in3] -> M195/3(E1)
  [in5] -> M195/4(T1)
  [in6] -> M195/5(EB1)
  [in13] -> M195/6(CT3)
  [in17] -> M195/7(T3)
  [in18] -> M195/8(EB3)
  M195/1(LL1) -> Eval194/1(In1)
  M195/2(LL3) -> Eval194/2(In3)
  Eval194/1(Out1) -> To Workspace194/1
  [in1] -> M196/1(CT1)
  [in2] -> M196/2(F1)
  [in3] -> M196/3(E1)
  [in5] -> M196/4(T1)
  [in6] -> M196/5(EB1)
  [in13] -> M196/6(CT3)
  [in17] -> M196/7(T3)
  [in18] -> M196/8(EB3)
  M196/1(LL1) -> Eval195/1(In1)
  M196/2(LL3) -> Eval195/2(In3)
  Eval195/1(Out1) -> To Workspace195/1
  [in1] -> M197/1(CT1)
  [in2] -> M197/2(F1)
  [in3] -> M197/3(E1)
  [in5] -> M197/4(T1)
  [in6] -> M197/5(EB1)
  [in13] -> M197/6(CT3)
  [in17] -> M197/7(T3)
  [in18] -> M197/8(EB3)
  M197/1(LL1) -> Eval196/1(In1)
  M197/2(LL3) -> Eval196/2(In3)
  Eval196/1(Out1) -> To Workspace196/1
  [in1] -> M198/1(CT1)
  [in2] -> M198/2(F1)
  [in3] -> M198/3(E1)
  [in5] -> M198/4(T1)
  [in6] -> M198/5(EB1)
  [in13] -> M198/6(CT3)
  [in17] -> M198/7(T3)
  [in18] -> M198/8(EB3)
  M198/1(LL1) -> Eval197/1(In1)
  M198/2(LL3) -> Eval197/2(In3)
  Eval197/1(Out1) -> To Workspace197/1
  [in1] -> M199/1(CT1)
  [in2] -> M199/2(F1)
  [in3] -> M199/3(E1)
  [in5] -> M199/4(T1)
  [in6] -> M199/5(EB1)
  [in13] -> M199/6(CT3)
  [in17] -> M199/7(T3)
  [in18] -> M199/8(EB3)
  M199/1(LL1) -> Eval198/1(In1)
  M199/2(LL3) -> Eval198/2(In3)
  Eval198/1(Out1) -> To Workspace198/1
  [in1] -> M222/1(CT1)
  [in2] -> M222/2(F1)
  [in3] -> M222/3(E1)
  [in5] -> M222/4(T1)
  [in6] -> M222/5(EB1)
  [in13] -> M222/6(CT3)
  [in17] -> M222/7(T3)
  [in18] -> M222/8(EB3)
  M222/1(LL1) -> Eval221/1(In1)
  M222/2(LL3) -> Eval221/2(In3)
  Eval221/1(Out1) -> To Workspace221/1
  [in1] -> M223/1(CT1)
  [in2] -> M223/2(F1)
  [in3] -> M223/3(E1)
  [in5] -> M223/4(T1)
  [in6] -> M223/5(EB1)
  [in13] -> M223/6(CT3)
  [in17] -> M223/7(T3)
  [in18] -> M223/8(EB3)
  M223/1(LL1) -> Eval222/1(In1)
  M223/2(LL3) -> Eval222/2(In3)
  Eval222/1(Out1) -> To Workspace222/1
  [in1] -> M224/1(CT1)
  [in2] -> M224/2(F1)
  [in3] -> M224/3(E1)
  [in5] -> M224/4(T1)
  [in6] -> M224/5(EB1)
  [in13] -> M224/6(CT3)
  [in17] -> M224/7(T3)
  [in18] -> M224/8(EB3)
  M224/1(LL1) -> Eval223/1(In1)
  M224/2(LL3) -> Eval223/2(In3)
  Eval223/1(Out1) -> To Workspace223/1
  [in1] -> M225/1(CT1)
  [in2] -> M225/2(F1)
  [in3] -> M225/3(E1)
  [in5] -> M225/4(T1)
  [in6] -> M225/5(EB1)
  [in13] -> M225/6(CT3)
  [in17] -> M225/7(T3)
  [in18] -> M225/8(EB3)
  M225/1(LL1) -> Eval224/1(In1)
  M225/2(LL3) -> Eval224/2(In3)
  Eval224/1(Out1) -> To Workspace224/1
  [in1] -> M226/1(CT1)
  [in2] -> M226/2(F1)
  [in3] -> M226/3(E1)
  [in5] -> M226/4(T1)
  [in6] -> M226/5(EB1)
  [in13] -> M226/6(CT3)
  [in17] -> M226/7(T3)
  [in18] -> M226/8(EB3)
  M226/1(LL1) -> Eval225/1(In1)
  M226/2(LL3) -> Eval225/2(In3)
  Eval225/1(Out1) -> To Workspace225/1
  [in1] -> M227/1(CT1)
  [in2] -> M227/2(F1)
  [in3] -> M227/3(E1)
  [in5] -> M227/4(T1)
  [in6] -> M227/5(EB1)
  [in13] -> M227/6(CT3)
  [in17] -> M227/7(T3)
  [in18] -> M227/8(EB3)
  M227/1(LL1) -> Eval226/1(In1)
  M227/2(LL3) -> Eval226/2(In3)
  Eval226/1(Out1) -> To Workspace226/1
  [in1] -> M228/1(CT1)
  [in2] -> M228/2(F1)
  [in3] -> M228/3(E1)
  [in5] -> M228/4(T1)
  [in6] -> M228/5(EB1)
  [in13] -> M228/6(CT3)
  [in17] -> M228/7(T3)
  [in18] -> M228/8(EB3)
  M228/1(LL1) -> Eval227/1(In1)
  M228/2(LL3) -> Eval227/2(In3)
  Eval227/1(Out1) -> To Workspace227/1
  [in1] -> M229/1(CT1)
  [in2] -> M229/2(F1)
  [in3] -> M229/3(E1)
  [in5] -> M229/4(T1)
  [in6] -> M229/5(EB1)
  [in13] -> M229/6(CT3)
  [in17] -> M229/7(T3)
  [in18] -> M229/8(EB3)
  M229/1(LL1) -> Eval228/1(In1)
  M229/2(LL3) -> Eval228/2(In3)
  Eval228/1(Out1) -> To Workspace228/1
  [in1] -> M230/1(CT1)
  [in2] -> M230/2(F1)
  [in3] -> M230/3(E1)
  [in5] -> M230/4(T1)
  [in6] -> M230/5(EB1)
  [in13] -> M230/6(CT3)
  [in17] -> M230/7(T3)
  [in18] -> M230/8(EB3)
  M230/1(LL1) -> Eval229/1(In1)
  M230/2(LL3) -> Eval229/2(In3)
  Eval229/1(Out1) -> To Workspace229/1
  [in1] -> M231/1(CT1)
  [in2] -> M231/2(F1)
  [in3] -> M231/3(E1)
  [in5] -> M231/4(T1)
  [in6] -> M231/5(EB1)
  [in13] -> M231/6(CT3)
  [in17] -> M231/7(T3)
  [in18] -> M231/8(EB3)
  M231/1(LL1) -> Eval230/1(In1)
  M231/2(LL3) -> Eval230/2(In3)
  Eval230/1(Out1) -> To Workspace230/1
  [in1] -> M232/1(CT1)
  [in2] -> M232/2(F1)
  [in3] -> M232/3(E1)
  [in5] -> M232/4(T1)
  [in6] -> M232/5(EB1)
  [in13] -> M232/6(CT3)
  [in17] -> M232/7(T3)
  [in18] -> M232/8(EB3)
  M232/1(LL1) -> Eval231/1(In1)
  M232/2(LL3) -> Eval231/2(In3)
  Eval231/1(Out1) -> To Workspace231/1
  [in1] -> M233/1(CT1)
  [in2] -> M233/2(F1)
  [in3] -> M233/3(E1)
  [in5] -> M233/4(T1)
  [in6] -> M233/5(EB1)
  [in13] -> M233/6(CT3)
  [in17] -> M233/7(T3)
  [in18] -> M233/8(EB3)
  M233/1(LL1) -> Eval232/1(In1)
  M233/2(LL3) -> Eval232/2(In3)
  Eval232/1(Out1) -> To Workspace232/1
  [in1] -> M234/1(CT1)
  [in2] -> M234/2(F1)
  [in3] -> M234/3(E1)
  [in5] -> M234/4(T1)
  [in6] -> M234/5(EB1)
  [in13] -> M234/6(CT3)
  [in17] -> M234/7(T3)
  [in18] -> M234/8(EB3)
  M234/1(LL1) -> Eval233/1(In1)
  M234/2(LL3) -> Eval233/2(In3)
  Eval233/1(Out1) -> To Workspace233/1
  [in1] -> M235/1(CT1)
  [in2] -> M235/2(F1)
  [in3] -> M235/3(E1)
  [in5] -> M235/4(T1)
  [in6] -> M235/5(EB1)
  [in13] -> M235/6(CT3)
  [in17] -> M235/7(T3)
  [in18] -> M235/8(EB3)
  M235/1(LL1) -> Eval234/1(In1)
  M235/2(LL3) -> Eval234/2(In3)
  Eval234/1(Out1) -> To Workspace234/1
  [in1] -> M236/1(CT1)
  [in2] -> M236/2(F1)
  [in3] -> M236/3(E1)
  [in5] -> M236/4(T1)
  [in6] -> M236/5(EB1)
  [in13] -> M236/6(CT3)
  [in17] -> M236/7(T3)
  [in18] -> M236/8(EB3)
  M236/1(LL1) -> Eval235/1(In1)
  M236/2(LL3) -> Eval235/2(In3)
  Eval235/1(Out1) -> To Workspace235/1
  [in1] -> M237/1(CT1)
  [in2] -> M237/2(F1)
  [in3] -> M237/3(E1)
  [in5] -> M237/4(T1)
  [in6] -> M237/5(EB1)
  [in13] -> M237/6(CT3)
  [in17] -> M237/7(T3)
  [in18] -> M237/8(EB3)
  M237/1(LL1) -> Eval236/1(In1)
  M237/2(LL3) -> Eval236/2(In3)
  Eval236/1(Out1) -> To Workspace236/1
  [in1] -> M238/1(CT1)
  [in2] -> M238/2(F1)
  [in3] -> M238/3(E1)
  [in5] -> M238/4(T1)
  [in6] -> M238/5(EB1)
  [in13] -> M238/6(CT3)
  [in17] -> M238/7(T3)
  [in18] -> M238/8(EB3)
  M238/1(LL1) -> Eval237/1(In1)
  M238/2(LL3) -> Eval237/2(In3)
  Eval237/1(Out1) -> To Workspace237/1
  [in1] -> M239/1(CT1)
  [in2] -> M239/2(F1)
  [in3] -> M239/3(E1)
  [in5] -> M239/4(T1)
  [in6] -> M239/5(EB1)
  [in13] -> M239/6(CT3)
  [in17] -> M239/7(T3)
  [in18] -> M239/8(EB3)
  M239/1(LL1) -> Eval238/1(In1)
  M239/2(LL3) -> Eval238/2(In3)
  Eval238/1(Out1) -> To Workspace238/1
  [in1] -> M240/1(CT1)
  [in2] -> M240/2(F1)
  [in3] -> M240/3(E1)
  [in5] -> M240/4(T1)
  [in6] -> M240/5(EB1)
  [in13] -> M240/6(CT3)
  [in17] -> M240/7(T3)
  [in18] -> M240/8(EB3)
  M240/1(LL1) -> Eval239/1(In1)
  M240/2(LL3) -> Eval239/2(In3)
  Eval239/1(Out1) -> To Workspace239/1
  [in1] -> M241/1(CT1)
  [in2] -> M241/2(F1)
  [in3] -> M241/3(E1)
  [in5] -> M241/4(T1)
  [in6] -> M241/5(EB1)
  [in13] -> M241/6(CT3)
  [in17] -> M241/7(T3)
  [in18] -> M241/8(EB3)
  M241/1(LL1) -> Eval240/1(In1)
  M241/2(LL3) -> Eval240/2(In3)
  Eval240/1(Out1) -> To Workspace240/1
  [in1] -> M242/1(CT1)
  [in2] -> M242/2(F1)
  [in3] -> M242/3(E1)
  [in5] -> M242/4(T1)
  [in6] -> M242/5(EB1)
  [in13] -> M242/6(CT3)
  [in17] -> M242/7(T3)
  [in18] -> M242/8(EB3)
  M242/1(LL1) -> Eval241/1(In1)
  M242/2(LL3) -> Eval241/2(In3)
  Eval241/1(Out1) -> To Workspace241/1
  [in1] -> M243/1(CT1)
  [in2] -> M243/2(F1)
  [in3] -> M243/3(E1)
  [in5] -> M243/4(T1)
  [in6] -> M243/5(EB1)
  [in13] -> M243/6(CT3)
  [in17] -> M243/7(T3)
  [in18] -> M243/8(EB3)
  M243/1(LL1) -> Eval242/1(In1)
  M243/2(LL3) -> Eval242/2(In3)
  Eval242/1(Out1) -> To Workspace242/1
  [in1] -> M244/1(CT1)
  [in2] -> M244/2(F1)
  [in3] -> M244/3(E1)
  [in5] -> M244/4(T1)
  [in6] -> M244/5(EB1)
  [in13] -> M244/6(CT3)
  [in17] -> M244/7(T3)
  [in18] -> M244/8(EB3)
  M244/1(LL1) -> Eval243/1(In1)
  M244/2(LL3) -> Eval243/2(In3)
  Eval243/1(Out1) -> To Workspace243/1
  [in1] -> M245/1(CT1)
  [in2] -> M245/2(F1)
  [in3] -> M245/3(E1)
  [in5] -> M245/4(T1)
  [in6] -> M245/5(EB1)
  [in13] -> M245/6(CT3)
  [in17] -> M245/7(T3)
  [in18] -> M245/8(EB3)
  M245/1(LL1) -> Eval244/1(In1)
  M245/2(LL3) -> Eval244/2(In3)
  Eval244/1(Out1) -> To Workspace244/1
  [in1] -> M246/1(CT1)
  [in2] -> M246/2(F1)
  [in3] -> M246/3(E1)
  [in5] -> M246/4(T1)
  [in6] -> M246/5(EB1)
  [in13] -> M246/6(CT3)
  [in17] -> M246/7(T3)
  [in18] -> M246/8(EB3)
  M246/1(LL1) -> Eval245/1(In1)
  M246/2(LL3) -> Eval245/2(In3)
  Eval245/1(Out1) -> To Workspace245/1
  Inputs/1(CT1) -> dtc_CT1/1
  dtc_CT1/1 -> CPSUT/1(CT1), [in1]
  Inputs/2(F1) -> dtc_F1/1
  dtc_F1/1 -> CPSUT/2(F1), [in2]
  Inputs/3(E1) -> dtc_E1/1
  dtc_E1/1 -> CPSUT/3(E1), [in3]
  Inputs/4(T1) -> dtc_T1/1
  dtc_T1/1 -> CPSUT/4(T1), [in5]
  Inputs/5(EB1) -> dtc_EB1/1
  dtc_EB1/1 -> CPSUT/5(EB1), [in6]
  Inputs/6(CT3) -> dtc_CT3/1
  dtc_CT3/1 -> CPSUT/6(CT3), [in13]
  Inputs/7(T3) -> dtc_T3/1
  dtc_T3/1 -> CPSUT/7(T3), [in17]
  Inputs/8(EB3) -> dtc_EB3/1
  dtc_EB3/1 -> CPSUT/8(EB3), [in18]

== system c00014M_harness/CPSUT ==
  note: VALUES
      | ---------------------------------
      | ControlType = 1 | 2 | 3
      | FillTank = 0 | 1
      | EmptyTank = 0 | 1
      | ManualReference between 0 and 1
      | Tempreature between 0 and 100
      | EmergencyButton = 0 | 1
      | LiquidLevel between 0 and 1 (hmax)
  note: Inputs For Tank2
  note: NAMES
      | --------------------------------------------
      | CT1 = ControlType Tank 1
      | F1 = Fill Tank 1
      | E1 = Empty Tank 1
      | MR1 = Manual Reference Tank1
      | T1 = Temperature Tank 1
      | EB1 = Emergency Button Tank 1
      | LL1 = Liquid Level 1
  note: Inputs For Tank3
  note: Inputs For Tank1
  CT1 : Inport
  F1 : Inport  Port=2
  E1 : Inport  Port=3
  T1 : Inport  Port=4
  EB1 : Inport  Port=5
  CT3 : Inport  Port=6
  T3 : Inport  Port=7
  EB3 : Inport  Port=8
  Tank1 : Subsystem
  Tank3 : Subsystem
  LL1 : Outport
  LL3 : Outport  Port=2
  wires:
  EB1/1 -> Tank1/5(EB1)
  Tank3/1(LL3) -> LL3/1, Tank1/6(LL3)
  T1/1 -> Tank1/4(T1)
  Tank1/1(LL1) -> LL1/1, Tank3/4(LL1)
  F1/1 -> Tank1/2(F1)
  E1/1 -> Tank1/3(E1)
  CT3/1 -> Tank3/1(CT3)
  EB3/1 -> Tank3/3(EB3)
  T3/1 -> Tank3/2(T3)
  CT1/1 -> Tank1/1(CT1)

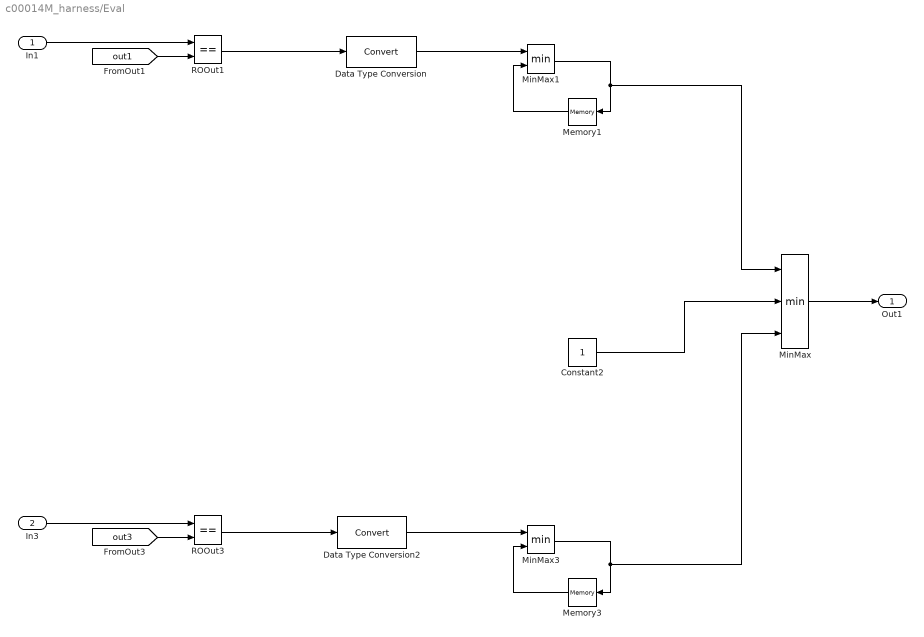
== system c00014M_harness/Eval ==
  In1 : Inport
  In3 : Inport  Port=2
  Constant2 : Constant
  Data Type Conversion : DataTypeConversion
  Data Type Conversion2 : DataTypeConversion
  Memory1 : Memory  InitialCondition=1
  Memory3 : Memory  InitialCondition=1
  MinMax : MinMax  Inputs=3
  MinMax1 : MinMax  Inputs=2
  MinMax3 : MinMax  Inputs=2
  ROOut1 : RelationalOperator  Operator===  OutDataTypeStr=boolean  RndMeth=Simplest
  ROOut3 : RelationalOperator  Operator===  OutDataTypeStr=boolean  RndMeth=Simplest
  Out1 : Outport
  wires:
  MinMax/1 -> Out1/1
  [out3] -> ROOut3/2
  In3/1 -> ROOut3/1
  [out1] -> ROOut1/2
  In1/1 -> ROOut1/1
  Memory1/1 -> MinMax1/2
  MinMax3/1 -> MinMax/3, Memory3/1
  ROOut3/1 -> Data Type Conversion2/1
  Memory3/1 -> MinMax3/2
  ROOut1/1 -> Data Type Conversion/1
  MinMax1/1 -> MinMax/1, Memory1/1
  Data Type Conversion/1 -> MinMax1/1
  Data Type Conversion2/1 -> MinMax3/1
  Constant2/1 -> MinMax/2

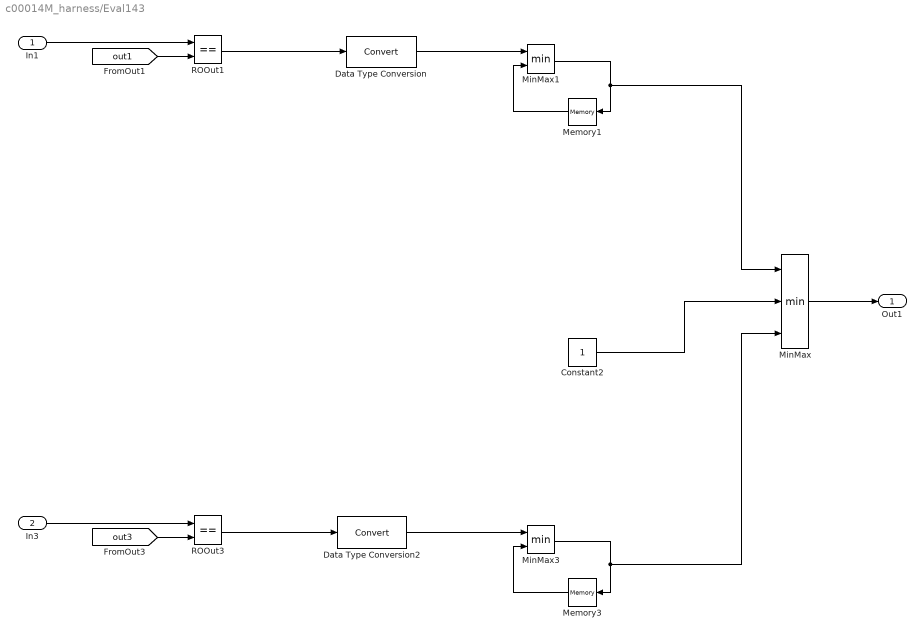
== system c00014M_harness/Eval143 ==
  In1 : Inport
  In3 : Inport  Port=2
  Constant2 : Constant
  Data Type Conversion : DataTypeConversion
  Data Type Conversion2 : DataTypeConversion
  Memory1 : Memory  InitialCondition=1
  Memory3 : Memory  InitialCondition=1
  MinMax : MinMax  Inputs=3
  MinMax1 : MinMax  Inputs=2
  MinMax3 : MinMax  Inputs=2
  ROOut1 : RelationalOperator  Operator===  OutDataTypeStr=boolean  RndMeth=Simplest
  ROOut3 : RelationalOperator  Operator===  OutDataTypeStr=boolean  RndMeth=Simplest
  Out1 : Outport
  wires:
  Data Type Conversion2/1 -> MinMax3/1
  Data Type Conversion/1 -> MinMax1/1
  MinMax1/1 -> Memory1/1, MinMax/1
  ROOut1/1 -> Data Type Conversion/1
  Memory3/1 -> MinMax3/2
  ROOut3/1 -> Data Type Conversion2/1
  MinMax3/1 -> Memory3/1, MinMax/3
  Memory1/1 -> MinMax1/2
  In1/1 -> ROOut1/1
  [out1] -> ROOut1/2
  In3/1 -> ROOut3/1
  [out3] -> ROOut3/2
  MinMax/1 -> Out1/1
  Constant2/1 -> MinMax/2

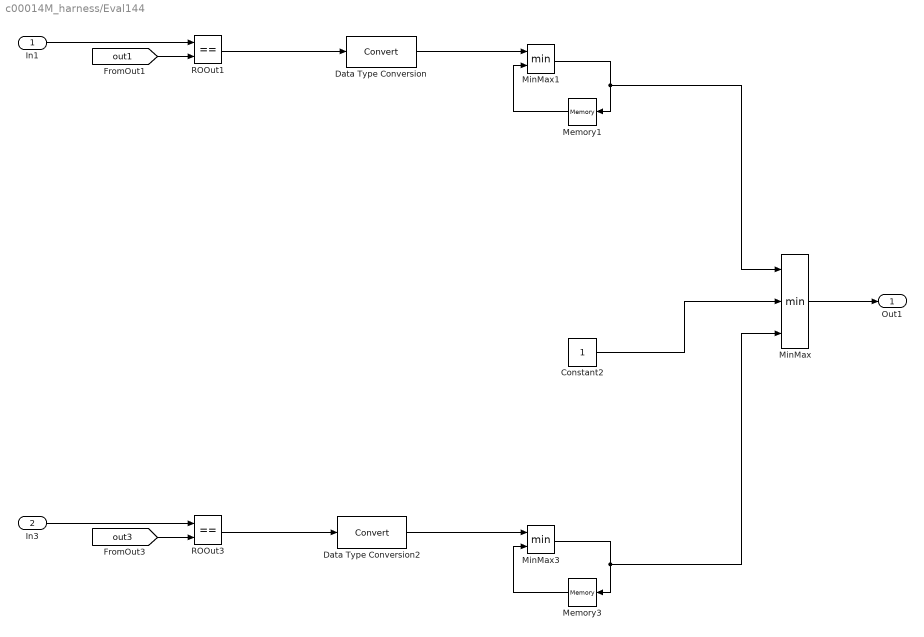
== system c00014M_harness/Eval144 ==
  In1 : Inport
  In3 : Inport  Port=2
  Constant2 : Constant
  Data Type Conversion : DataTypeConversion
  Data Type Conversion2 : DataTypeConversion
  Memory1 : Memory  InitialCondition=1
  Memory3 : Memory  InitialCondition=1
  MinMax : MinMax  Inputs=3
  MinMax1 : MinMax  Inputs=2
  MinMax3 : MinMax  Inputs=2
  ROOut1 : RelationalOperator  Operator===  OutDataTypeStr=boolean  RndMeth=Simplest
  ROOut3 : RelationalOperator  Operator===  OutDataTypeStr=boolean  RndMeth=Simplest
  Out1 : Outport
  wires:
  Data Type Conversion2/1 -> MinMax3/1
  Data Type Conversion/1 -> MinMax1/1
  MinMax1/1 -> Memory1/1, MinMax/1
  ROOut1/1 -> Data Type Conversion/1
  Memory3/1 -> MinMax3/2
  ROOut3/1 -> Data Type Conversion2/1
  MinMax3/1 -> Memory3/1, MinMax/3
  Memory1/1 -> MinMax1/2
  In1/1 -> ROOut1/1
  [out1] -> ROOut1/2
  In3/1 -> ROOut3/1
  [out3] -> ROOut3/2
  MinMax/1 -> Out1/1
  Constant2/1 -> MinMax/2

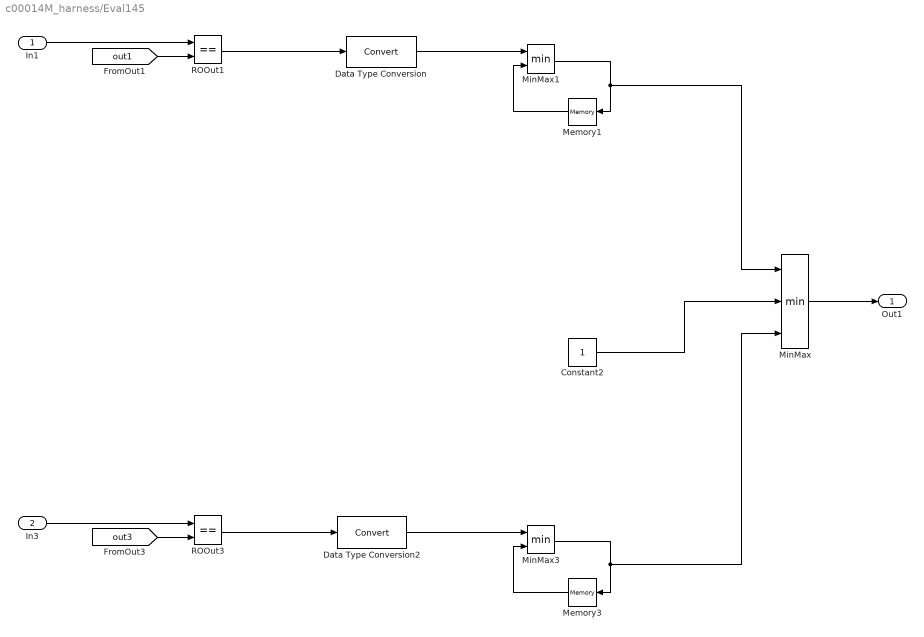
== system c00014M_harness/Eval145 ==
  In1 : Inport
  In3 : Inport  Port=2
  Constant2 : Constant
  Data Type Conversion : DataTypeConversion
  Data Type Conversion2 : DataTypeConversion
  Memory1 : Memory  InitialCondition=1
  Memory3 : Memory  InitialCondition=1
  MinMax : MinMax  Inputs=3
  MinMax1 : MinMax  Inputs=2
  MinMax3 : MinMax  Inputs=2
  ROOut1 : RelationalOperator  Operator===  OutDataTypeStr=boolean  RndMeth=Simplest
  ROOut3 : RelationalOperator  Operator===  OutDataTypeStr=boolean  RndMeth=Simplest
  Out1 : Outport
  wires:
  Data Type Conversion2/1 -> MinMax3/1
  Data Type Conversion/1 -> MinMax1/1
  MinMax1/1 -> Memory1/1, MinMax/1
  ROOut1/1 -> Data Type Conversion/1
  Memory3/1 -> MinMax3/2
  ROOut3/1 -> Data Type Conversion2/1
  MinMax3/1 -> Memory3/1, MinMax/3
  Memory1/1 -> MinMax1/2
  In1/1 -> ROOut1/1
  [out1] -> ROOut1/2
  In3/1 -> ROOut3/1
  [out3] -> ROOut3/2
  MinMax/1 -> Out1/1
  Constant2/1 -> MinMax/2

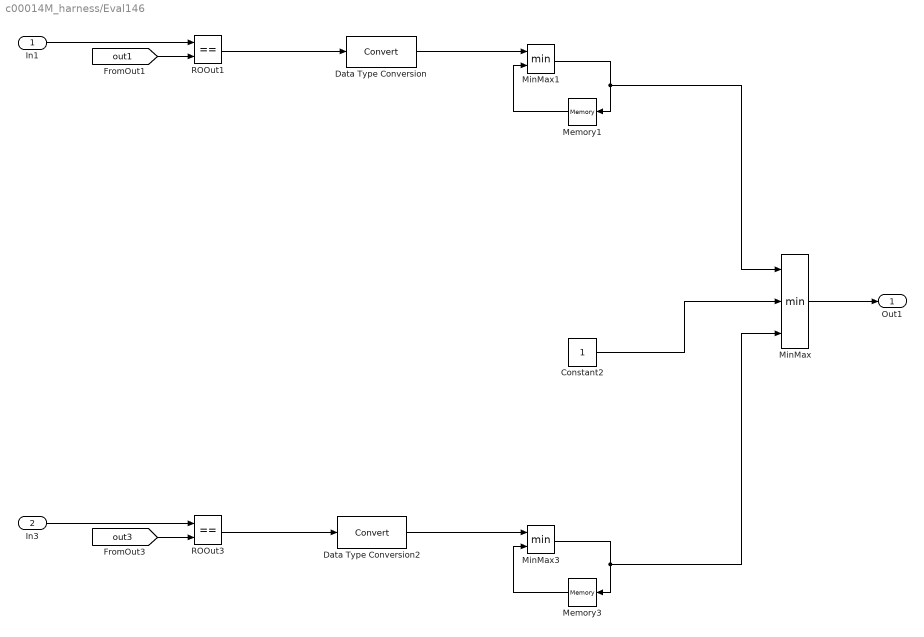
== system c00014M_harness/Eval146 ==
  In1 : Inport
  In3 : Inport  Port=2
  Constant2 : Constant
  Data Type Conversion : DataTypeConversion
  Data Type Conversion2 : DataTypeConversion
  Memory1 : Memory  InitialCondition=1
  Memory3 : Memory  InitialCondition=1
  MinMax : MinMax  Inputs=3
  MinMax1 : MinMax  Inputs=2
  MinMax3 : MinMax  Inputs=2
  ROOut1 : RelationalOperator  Operator===  OutDataTypeStr=boolean  RndMeth=Simplest
  ROOut3 : RelationalOperator  Operator===  OutDataTypeStr=boolean  RndMeth=Simplest
  Out1 : Outport
  wires:
  Data Type Conversion2/1 -> MinMax3/1
  Data Type Conversion/1 -> MinMax1/1
  MinMax1/1 -> Memory1/1, MinMax/1
  ROOut1/1 -> Data Type Conversion/1
  Memory3/1 -> MinMax3/2
  ROOut3/1 -> Data Type Conversion2/1
  MinMax3/1 -> Memory3/1, MinMax/3
  Memory1/1 -> MinMax1/2
  In1/1 -> ROOut1/1
  [out1] -> ROOut1/2
  In3/1 -> ROOut3/1
  [out3] -> ROOut3/2
  MinMax/1 -> Out1/1
  Constant2/1 -> MinMax/2

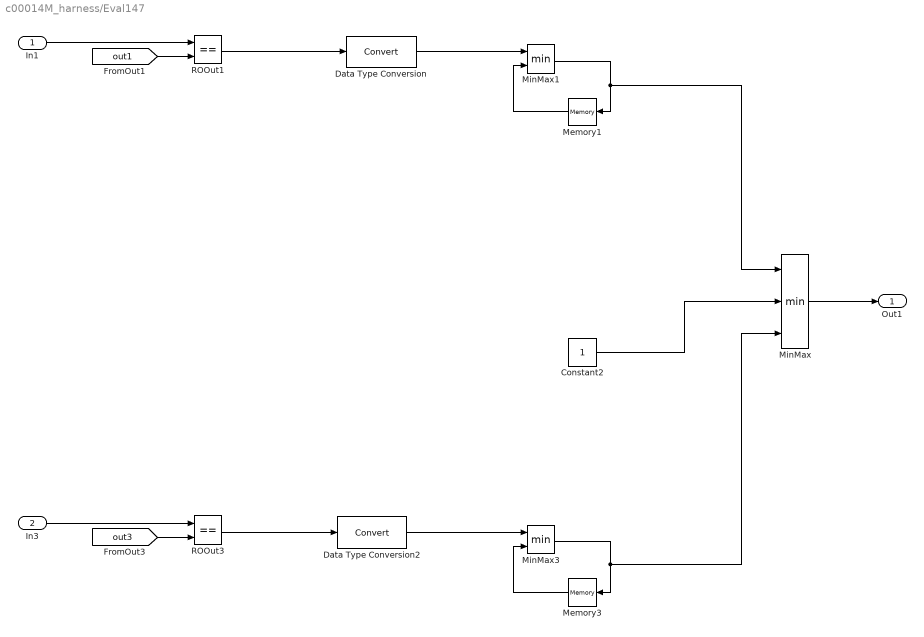
== system c00014M_harness/Eval147 ==
  In1 : Inport
  In3 : Inport  Port=2
  Constant2 : Constant
  Data Type Conversion : DataTypeConversion
  Data Type Conversion2 : DataTypeConversion
  Memory1 : Memory  InitialCondition=1
  Memory3 : Memory  InitialCondition=1
  MinMax : MinMax  Inputs=3
  MinMax1 : MinMax  Inputs=2
  MinMax3 : MinMax  Inputs=2
  ROOut1 : RelationalOperator  Operator===  OutDataTypeStr=boolean  RndMeth=Simplest
  ROOut3 : RelationalOperator  Operator===  OutDataTypeStr=boolean  RndMeth=Simplest
  Out1 : Outport
  wires:
  Data Type Conversion2/1 -> MinMax3/1
  Data Type Conversion/1 -> MinMax1/1
  MinMax1/1 -> Memory1/1, MinMax/1
  ROOut1/1 -> Data Type Conversion/1
  Memory3/1 -> MinMax3/2
  ROOut3/1 -> Data Type Conversion2/1
  MinMax3/1 -> Memory3/1, MinMax/3
  Memory1/1 -> MinMax1/2
  In1/1 -> ROOut1/1
  [out1] -> ROOut1/2
  In3/1 -> ROOut3/1
  [out3] -> ROOut3/2
  MinMax/1 -> Out1/1
  Constant2/1 -> MinMax/2

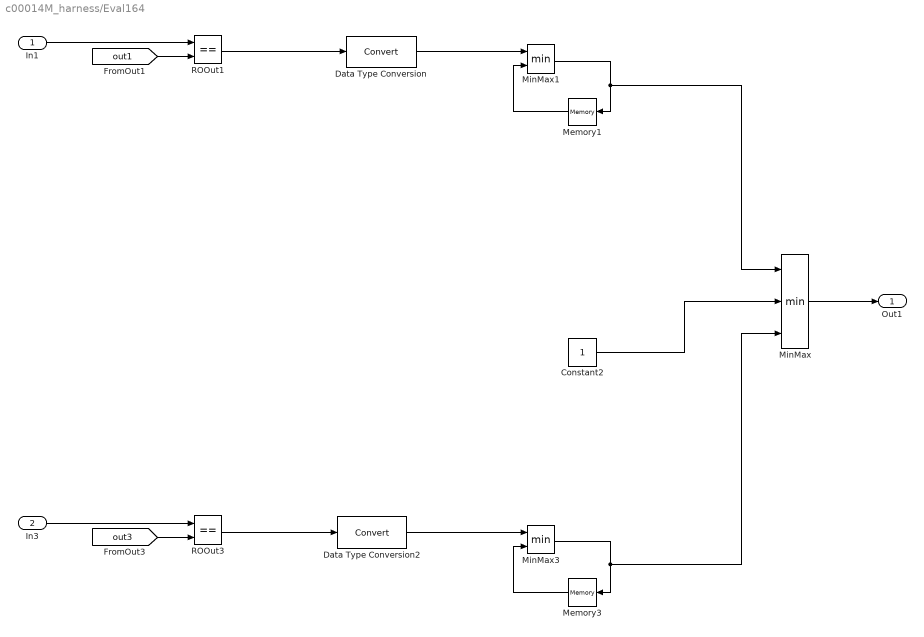
== system c00014M_harness/Eval164 ==
  In1 : Inport
  In3 : Inport  Port=2
  Constant2 : Constant
  Data Type Conversion : DataTypeConversion
  Data Type Conversion2 : DataTypeConversion
  Memory1 : Memory  InitialCondition=1
  Memory3 : Memory  InitialCondition=1
  MinMax : MinMax  Inputs=3
  MinMax1 : MinMax  Inputs=2
  MinMax3 : MinMax  Inputs=2
  ROOut1 : RelationalOperator  Operator===  OutDataTypeStr=boolean  RndMeth=Simplest
  ROOut3 : RelationalOperator  Operator===  OutDataTypeStr=boolean  RndMeth=Simplest
  Out1 : Outport
  wires:
  Data Type Conversion2/1 -> MinMax3/1
  Data Type Conversion/1 -> MinMax1/1
  MinMax1/1 -> Memory1/1, MinMax/1
  ROOut1/1 -> Data Type Conversion/1
  Memory3/1 -> MinMax3/2
  ROOut3/1 -> Data Type Conversion2/1
  MinMax3/1 -> Memory3/1, MinMax/3
  Memory1/1 -> MinMax1/2
  In1/1 -> ROOut1/1
  [out1] -> ROOut1/2
  In3/1 -> ROOut3/1
  [out3] -> ROOut3/2
  MinMax/1 -> Out1/1
  Constant2/1 -> MinMax/2

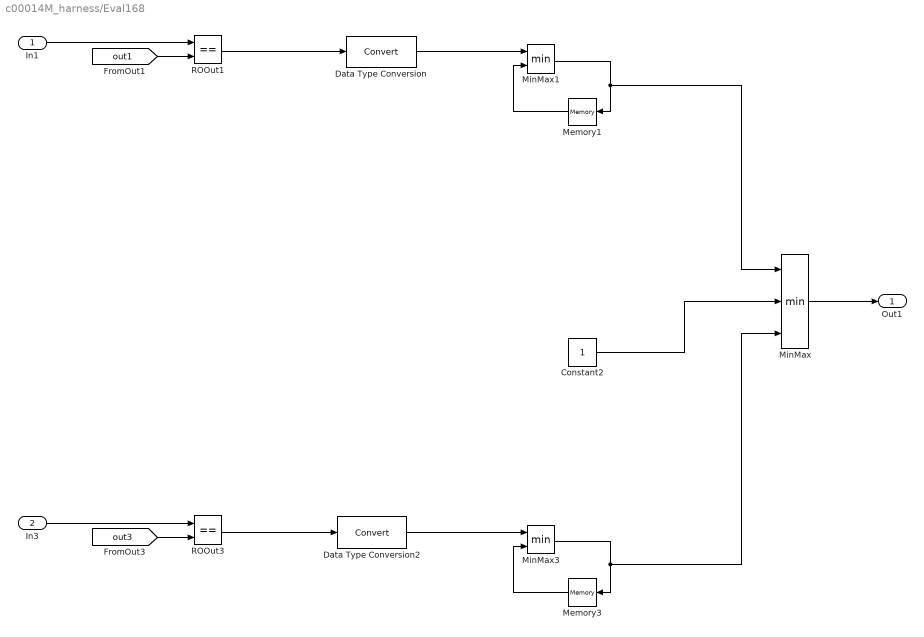
== system c00014M_harness/Eval168 ==
  In1 : Inport
  In3 : Inport  Port=2
  Constant2 : Constant
  Data Type Conversion : DataTypeConversion
  Data Type Conversion2 : DataTypeConversion
  Memory1 : Memory  InitialCondition=1
  Memory3 : Memory  InitialCondition=1
  MinMax : MinMax  Inputs=3
  MinMax1 : MinMax  Inputs=2
  MinMax3 : MinMax  Inputs=2
  ROOut1 : RelationalOperator  Operator===  OutDataTypeStr=boolean  RndMeth=Simplest
  ROOut3 : RelationalOperator  Operator===  OutDataTypeStr=boolean  RndMeth=Simplest
  Out1 : Outport
  wires:
  Data Type Conversion2/1 -> MinMax3/1
  Data Type Conversion/1 -> MinMax1/1
  MinMax1/1 -> Memory1/1, MinMax/1
  ROOut1/1 -> Data Type Conversion/1
  Memory3/1 -> MinMax3/2
  ROOut3/1 -> Data Type Conversion2/1
  MinMax3/1 -> Memory3/1, MinMax/3
  Memory1/1 -> MinMax1/2
  In1/1 -> ROOut1/1
  [out1] -> ROOut1/2
  In3/1 -> ROOut3/1
  [out3] -> ROOut3/2
  MinMax/1 -> Out1/1
  Constant2/1 -> MinMax/2
